simulink model "continuous_smith"  (R2017a)
settings: Solver=VariableStepAuto  StartTime=0.0  StopTime=20.0  RelTol=1e-3
settings Model: Creator=aous  LastModifiedBy=aous

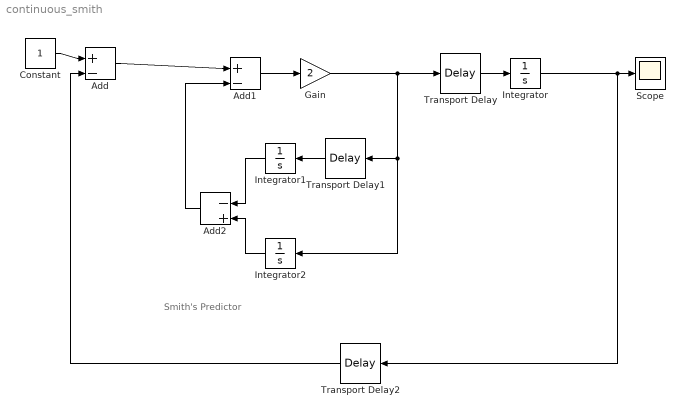
== system continuous_smith ==
  note: Smith's Predictor
  Add : Sum  Inputs=+|-
  Add1 : Sum  Inputs=+|-
  Add2 : Sum  Inputs=-|+
  Constant : Constant
  Gain : Gain  Gain=2
  Integrator : Integrator
  Integrator1 : Integrator
  Integrator2 : Integrator
  Scope : Scope
  Transport Delay : TransportDelay
  Transport Delay1 : TransportDelay  DelayTime=2
  Transport Delay2 : TransportDelay
  wires:
  Add/1 -> Add1/1
  Transport Delay/1 -> Integrator/1
  Integrator/1 -> Transport Delay2/1, Scope/1
  Constant/1 -> Add/1
  Gain/1 -> Integrator2/1, Transport Delay1/1, Transport Delay/1
  Add1/1 -> Gain/1
  Add2/1 -> Add1/2
  Transport Delay1/1 -> Integrator1/1
  Integrator1/1 -> Add2/1
  Integrator2/1 -> Add2/2
  Transport Delay2/1 -> Add/2
